simulink model "FMsendrec"  (Simulink 9.0)
settings: Solver=FixedStepDiscrete  StartTime=0.0  StopTime=1000  RelTol=1e-3
PreLoadFcn:
  | setenv('MW_MINGW64_LOC','C:\TDM-GCC-64')
StartFcn:
  | tic
StopFcn:
  | toc;
libraries: UN_HIL_Lib x2, dspobslib x1
Description:
  | QPSK Transmitter and Receiver.
  | 
  | This model shows the implementation of a QPSK transmitter and receiver.
settings Model: FPTRunName=Active  Creator=The MathWorks Inc.  LastModifiedBy=Administrator
settings DataIOCC: LimitDataPoints=on  SignalLoggingSaveFormat=ModelDataLogs  SaveOutput=off  SaveTime=off
settings OptimizationCC: BooleanDataType=off  DefaultParameterBehavior=Inlined  ExpressionDepthLimit=2147483647  LocalBlockOutputs=off
settings DebuggingCC: AlgebraicLoopMsg=error  SolverPrmCheckMsg=warning  SingleTaskRateTransMsg=error  ParameterPrecisionLossMsg=none  FcnCallInpInsideContextMsg=warning  StateNameClashWarn=warning
settings HardwareCC: TargetBitPerPointer=64  TargetBitPerSizeT=64  TargetBitPerPtrDiffT=64  TargetLongLongMode=on  TargetIntDivRoundTo=Zero  TargetEndianess=LittleEndian  TargetWordSize=64  TargetHWDeviceType=Generic->MATLAB Host Computer  ProdEqTarget=off
settings GRTTargetCC: GeneratePreprocessorConditionals=Disable all
settings ConfigComp: CovSFcnEnable=off
settings SimEventsCC: propDiagStatOutput=1  propPreventDuplicateEvents=0

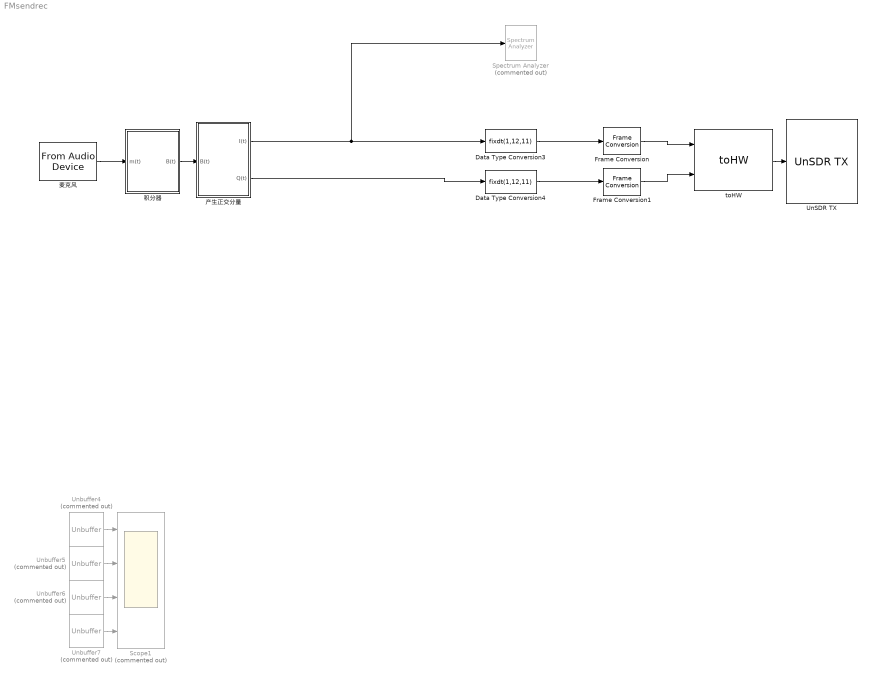
== system FMsendrec ==
  Data Type Conversion3 : DataTypeConversion  OutDataTypeStr=fixdt(1,12,11)
  Data Type Conversion4 : DataTypeConversion  OutDataTypeStr=fixdt(1,12,11)
  Frame Conversion : FrameConversion  InheritSamplingMode=off  OutFrame=Sample-based
  Frame Conversion1 : FrameConversion  InheritSamplingMode=off  OutFrame=Sample-based
  Scope1 : Scope  Commented=on  NumInputPorts=4
  Spectrum Analyzer : SpectrumAnalyzer  Commented=on
  UnSDR TX : UN_HIL_Lib/UnSDR TX  SystemSampleTime=-1
      settings: SourceProductName=HIL Blockset
  Unbuffer{4..7} (4 alike) : Unbuffer  Commented=on
  toHW : UN_HIL_Lib/toHW  SystemSampleTime=-1
      settings: SourceProductName=HIL Blockset
  产生正交分量 : Subsystem
  积分器 : Subsystem
  麦克风 : dspobslib/From Audio Device  deviceName=Default  numChannels=1  sampleRate=128000  deviceDatatype=Determine from output data type  autoBufferSize=on  bufferSize=4096  queueDuration=1.0  frameSize=1  outputDatatype=single  defaultInputChannelMapping=on  inputChannelMapping=1:2  outputNumOverrunSamples=off  OutputFrames=on
      settings: SourceProductName=DSP System Toolbox  SourceProductBaseCode=DS
  wires:
  Unbuffer5/1 -> Scope1/2
  Unbuffer6/1 -> Scope1/3
  Unbuffer7/1 -> Scope1/4
  Unbuffer4/1 -> Scope1/1
  Data Type Conversion3/1 -> Frame Conversion/1
  Data Type Conversion4/1 -> Frame Conversion1/1
  Frame Conversion1/1 -> toHW/2
  Frame Conversion/1 -> toHW/1
  麦克风/1 -> 积分器/1(m(t))
  积分器/1(B(t)) -> 产生正交分量/1(B(t))
  产生正交分量/1(I(t)) -> Data Type Conversion3/1, Spectrum Analyzer/1
  产生正交分量/2(Q(t)) -> Data Type Conversion4/1
  toHW/1 -> UnSDR TX/1

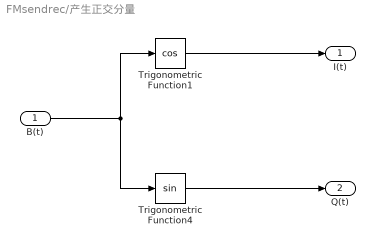
== system FMsendrec/产生正交分量 ==
  B(t) : Inport
  Trigonometric Function1 : Trigonometry  Operator=cos  NumberOfIterations=16
  Trigonometric Function4 : Trigonometry  NumberOfIterations=16
  I(t) : Outport
  Q(t) : Outport  Port=2
  wires:
  Trigonometric Function1/1 -> I(t)/1
  B(t)/1 -> Trigonometric Function4/1, Trigonometric Function1/1
  Trigonometric Function4/1 -> Q(t)/1

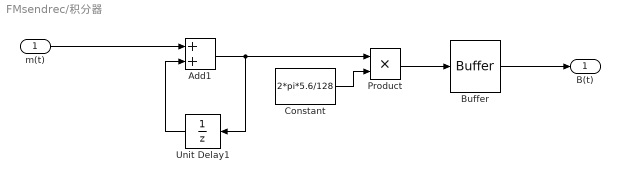
== system FMsendrec/积分器 ==
  m(t) : Inport
  Add1 : Sum  OutDataTypeStr=Inherit: Same as first input
  Buffer : Buffer  N=4096
  Constant : Constant  Value=2*pi*5.6/128  VectorParams1D=off  SampleTime=-1
  Product : Product  RndMeth=Zero  OutDataTypeStr=Inherit: Same as first input
  Unit Delay1 : UnitDelay  SampleTime=-1
  B(t) : Outport
  wires:
  Product/1 -> Buffer/1
  Constant/1 -> Product/2
  Add1/1 -> Product/1, Unit Delay1/1
  Unit Delay1/1 -> Add1/2
  m(t)/1 -> Add1/1
  Buffer/1 -> B(t)/1
